simulink model "Pcontroller"  (R2021b)
settings: Solver=VariableStepAuto  StartTime=0.0  StopTime=20  RelTol=1e-3
model workspace (MAT data in the model file):
  L = 0.2
values from neighbouring files (symbols this model uses):
  g = 9.81    [simConstants.m]
  Td = 10e-6    (= 1e-05)    [simConstants.m]
  theta0 = deg2rad(5)    [simConstants.m]
libraries: simulink_extras x1, slpidlib x1
settings Model: Creator=logan  LastModifiedBy=logan

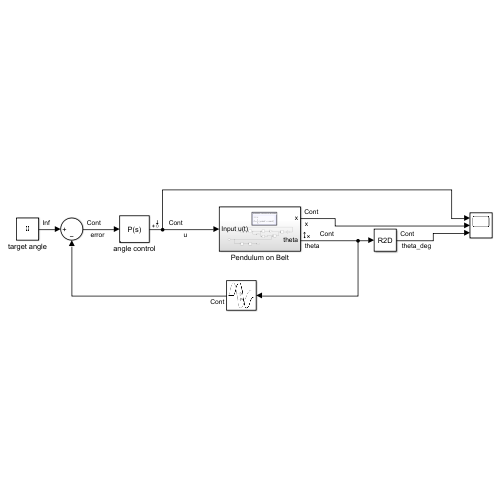
[thumbnail: Simulink's stored preview of the top-level diagram]
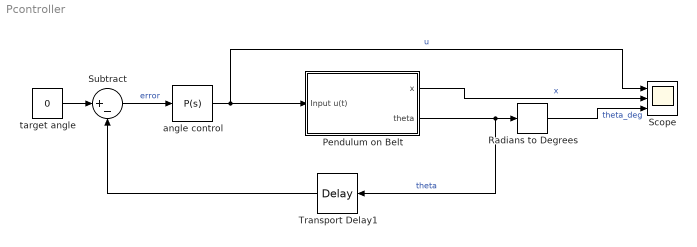
== system Pcontroller ==
  Pendulum on Belt : Subsystem
  Radians to Degrees : simulink_extras/Transformations/Radians to Degrees
  Scope : Scope  NumInputPorts=3
  Subtract : Sum  Inputs=|+-
  Transport Delay1 : TransportDelay  DelayTime=Td  InitialOutput=theta0
  angle control : slpidlib/PID Controller  Controller=P  Form=Parallel  TimeDomain=Continuous-time  UseExternalTs=off  SampleTime=-1  IntegratorMethod=Forward Euler  FilterMethod=Forward Euler  ControllerParametersSource=internal  P=-10  I=0  D=0  UseFilter=on  N=100  TunerSelectOption=Transfer Function Based (PID Tuner App)  InitialConditionSource=internal  InitialConditionForIntegrator=0  InitialConditionForFilter=0  DifferentiatorICPrevScaledInput=0  ExternalReset=none  TrackingMode=off  Kt=1  LimitOutput=off  SatLimitsSource=internal  UpperSaturationLimit=inf  LowerSaturationLimit=-inf  LinearizeAsGain=on  AntiWindupMode=none  Kb=1  POutMin=[]  POutMax=[]  IOutMin=[]  IOutMax=[]  DOutMin=[]  DOutMax=[]  NOutMin=[]  NOutMax=[]  SumOutMin=[]  SumOutMax=[]  SaturationOutMin=[]  SaturationOutMax=[]  PParamMin=[]  PParamMax=[]  IParamMin=[]  IParamMax=[]  DParamMin=[]  DParamMax=[]  NParamMin=[]  NParamMax=[]  KbParamMin=[]  KbParamMax=[]  KtParamMin=[]  KtParamMax=[]  KbOutMin=[]  KbOutMax=[]  KtOutMin=[]  KtOutMax=[]  IntegratorOutMin=[]  IntegratorOutMax=[]  FilterOutMin=[]  FilterOutMax=[]  SumI1OutMin=[]  SumI1OutMax=[]  SumI2OutMin=[]  SumI2OutMax=[]  SumI3OutMin=[]  SumI3OutMax=[]  SumI4OutMin=[]  SumI4OutMax=[]  SumDOutMin=[]  SumDOutMax=[]  DifferentiatorOutMin=[]  DifferentiatorOutMax=[]  FilterDiffOutCoefMin=[]  FilterDiffOutCoefMax=[]  ReciprocalOutMin=[]  ReciprocalOutMax=[]  SumDenOutMin=[]  SumDenOutMax=[]  SumNumOutMin=[]  SumNumOutMax=[]  DivideOutMin=[]  DivideOutMax=[]  UdiffTsProdOutMin=[]  UdiffTsProdOutMax=[]  NTsProdOutMin=[]  NTsProdOutMax=[]  UintegralTsProdOutMin=[]  UintegralTsProdOutMax=[]  UngainTsProdOutMin=[]  UngainTsProdOutMax=[]  IntegratorContinuousStateAttributes=''  IntegratorStateMustResolveToSignalObject=off  IntegratorRTWStateStorageClass=Auto  FilterContinuousStateAttributes=''  FilterStateMustResolveToSignalObject=off  FilterRTWStateStorageClass=Auto  ParallelPVariant=InternalParameters  IdealPVariant=Disabled  IVariant=Disabled  DVariant=Disabled  IntegratorVariant=Disabled  SatVariant=Disabled  AWVariant=Disabled  PCopyVariant=Disabled  TRVariant=Disabled  FdbkBlocksVariant=Forward  IdealPFdbkVariant=Disabled  SatFdbkVariant=Disabled  DerivativeFilterVariant=Disabled  NVariant=Disabled  NCopyVariant=Disabled_SignalSpec  FilterICVariant=Disabled  IntegratorICVariant=Disabled  ExternalResetVariant=Disabled  TRSumVariant=Passthrough  SumFdbkVariant=Disabled  SumVariant=Passthrough_P  TsampFilterVariant=InternalTs  TsampNgainVariant=Passthrough  TsampIntegralVariant=Disabled_SignalSpec  ExternalSaturationOutDataTypeStr=Inherit: Same as second input
  target angle : Constant  Value=0  OutDataTypeStr=Inherit: Inherit via back propagation
  wires:
  Pendulum on Belt/1(x) -> Scope/2  "x"
  Pendulum on Belt/2(theta) -> Transport Delay1/1, Radians to Degrees/1  "theta"
  Radians to Degrees/1 -> Scope/3  "theta_deg"
  angle control/1 -> Pendulum on Belt/1(Input u(t)), Scope/1  "u"
  Transport Delay1/1 -> Subtract/2
  Subtract/1 -> angle control/1  "error"
  target angle/1 -> Subtract/1

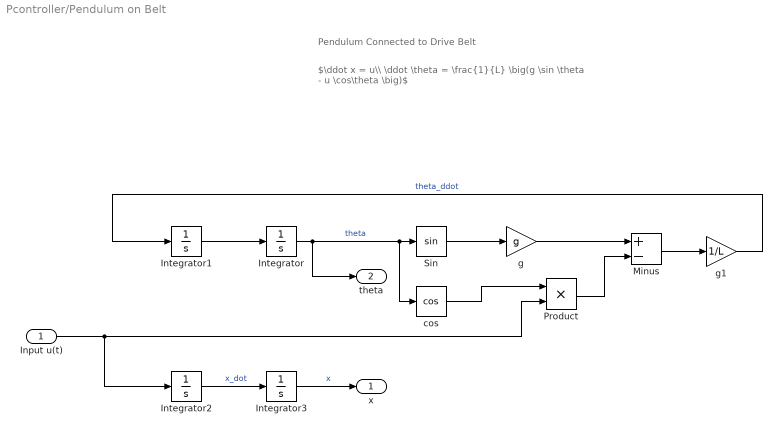
== system Pcontroller/Pendulum on Belt ==
  note: Pendulum Connected to Drive Belt
  note: $\ddot x = u\\ \ddot \theta = \frac{1}{L} \big(g \sin \theta - u \cos\theta \big)$
  Input u(t) : Inport
  Integrator : Integrator  InitialCondition=theta0
  Integrator1 : Integrator
  Integrator2 : Integrator
  Integrator3 : Integrator
  Minus : Sum  Inputs=+-
  Product : Product
  Sin : Trigonometry
  cos : Trigonometry  Operator=cos
  g : Gain  Gain=g
  g1 : Gain  Gain=1/L
  x : Outport
  theta : Outport  Port=2
  wires:
  Integrator/1 -> theta/1, cos/1, Sin/1  "theta"
  Integrator1/1 -> Integrator/1
  Input u(t)/1 -> Integrator2/1, Product/2
  g/1 -> Minus/1
  Sin/1 -> g/1
  cos/1 -> Product/1
  Integrator3/1 -> x/1  "x"
  Product/1 -> Minus/2
  Minus/1 -> g1/1
  g1/1 -> Integrator1/1  "theta_ddot"
  Integrator2/1 -> Integrator3/1  "x_dot"
